simulink model "a1e2"  (R2020a)
settings: Solver=VariableStepAuto  StartTime=0.0  StopTime=50  RelTol=1e-3
settings Model: Creator=vivek vivian  LastModifiedBy=vivek vivian

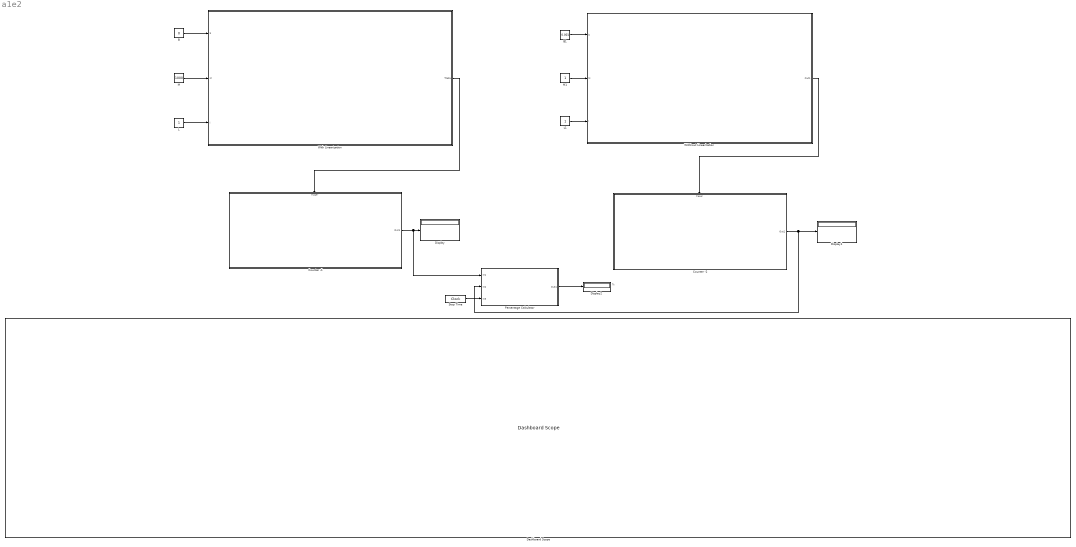
== system a1e2 ==
  note: %
  B : Constant  Value=0
  B1 : Constant  Value=0.001
  Counter -1 : Subsystem
  Counter -2 : Subsystem
  Dashboard Scope : DashboardScope
  Display : Display
  Display1 : Display
  Display2 : Display
  L : Constant
  L1 : Constant
  M : Constant  Value=1000
  M1 : Constant
  Percentage Calculator : Subsystem
  Stop Time : DigitalClock
  With Linearization : Subsystem
  Withhout Linearization : Subsystem
  wires:
  Counter -1/1(Out1) -> Percentage Calculator/1(In1), Display/1
  With Linearization/1(Theta) -> Counter -1/Trigger
  Counter -2/1(Out1) -> Percentage Calculator/2(In2), Display1/1
  Withhout Linearization/1(Out1) -> Counter -2/Trigger
  Percentage Calculator/1(Out1) -> Display2/1
  B/1 -> With Linearization/1(b)
  M/1 -> With Linearization/2(M)
  L/1 -> With Linearization/3(l)
  L1/1 -> Withhout Linearization/3(l)
  M1/1 -> Withhout Linearization/2(M)
  B1/1 -> Withhout Linearization/1(b)
  Stop Time/1 -> Percentage Calculator/3(In3)

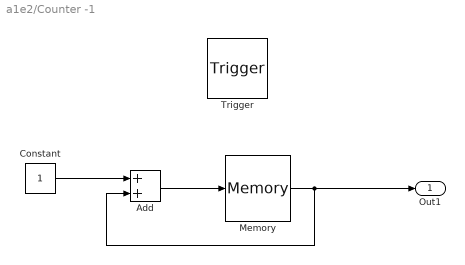
== system a1e2/Counter -1 ==
  Trigger : TriggerPort  VariantControl=Variant  PortDimensions=1
  Add : Sum
  Constant : Constant
  Memory : Memory  InheritSampleTime=on
  Out1 : Outport
  wires:
  Constant/1 -> Add/1
  Add/1 -> Memory/1
  Memory/1 -> Add/2, Out1/1

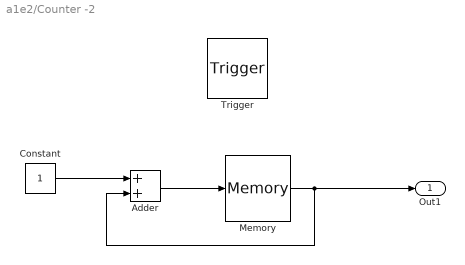
== system a1e2/Counter -2 ==
  Trigger : TriggerPort  VariantControl=Variant  PortDimensions=1
  Adder : Sum
  Constant : Constant
  Memory : Memory  InheritSampleTime=on
  Out1 : Outport
  wires:
  Constant/1 -> Adder/1
  Adder/1 -> Memory/1
  Memory/1 -> Adder/2, Out1/1

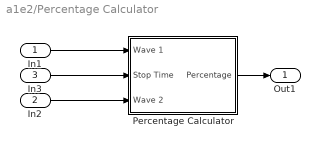
== system a1e2/Percentage Calculator ==
  In1 : Inport
  In2 : Inport  Port=2
  In3 : Inport  Port=3
  Percentage Calculator : Subsystem
  Out1 : Outport
  wires:
  In1/1 -> Percentage Calculator/1(Wave 1)
  In3/1 -> Percentage Calculator/2(Stop Time)
  In2/1 -> Percentage Calculator/3(Wave 2)
  Percentage Calculator/1(Percentage) -> Out1/1

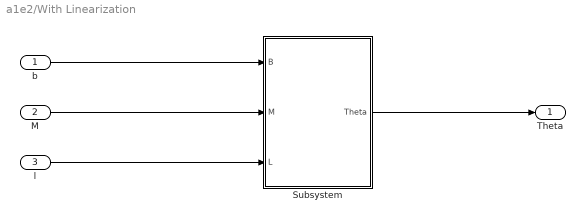
== system a1e2/With Linearization ==
  b : Inport
  M : Inport  Port=2
  l : Inport  Port=3
  Subsystem : Subsystem
  Theta : Outport
  wires:
  b/1 -> Subsystem/1(B)
  M/1 -> Subsystem/2(M)
  l/1 -> Subsystem/3(L)
  Subsystem/1(Theta) -> Theta/1

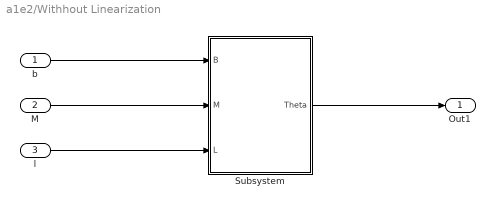
== system a1e2/Withhout Linearization ==
  b : Inport
  M : Inport  Port=2
  l : Inport  Port=3
  Subsystem : Subsystem
  Out1 : Outport
  wires:
  b/1 -> Subsystem/1(B)
  M/1 -> Subsystem/2(M)
  l/1 -> Subsystem/3(L)
  Subsystem/1(Theta) -> Out1/1

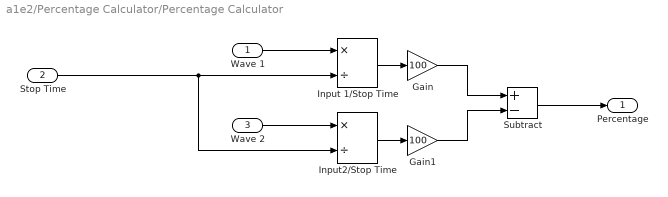
== system a1e2/Percentage Calculator/Percentage Calculator ==
  Wave 1 : Inport
  Stop Time : Inport  Port=2
  Wave 2 : Inport  Port=3
  Gain : Gain  Gain=100
  Gain1 : Gain  Gain=100
  Input 1/Stop Time : Product  Inputs=*/
  Input2/Stop Time : Product  Inputs=*/
  Subtract : Sum  Inputs=+-
  Percentage : Outport
  wires:
  Input 1/Stop Time/1 -> Gain/1
  Input2/Stop Time/1 -> Gain1/1
  Stop Time/1 -> Input2/Stop Time/2, Input 1/Stop Time/2
  Subtract/1 -> Percentage/1
  Gain1/1 -> Subtract/2
  Wave 2/1 -> Input2/Stop Time/1
  Wave 1/1 -> Input 1/Stop Time/1
  Gain/1 -> Subtract/1

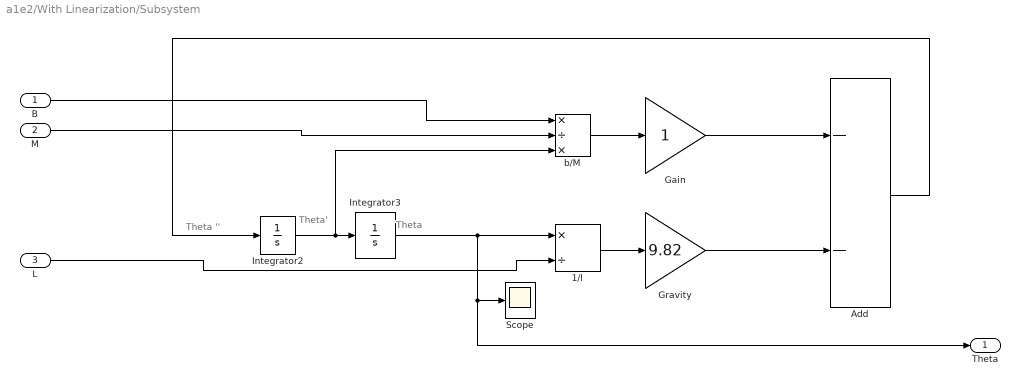
== system a1e2/With Linearization/Subsystem ==
  note: Theta
  note: Theta'
  note: Theta ''
  B : Inport
  M : Inport  Port=2
  L : Inport  Port=3
  1/l : Product  Inputs=*/
  Add : Sum  Inputs=--
  Gain : Gain
  Gravity : Gain  Gain=9.82
  Integrator2 : Integrator
  Integrator3 : Integrator  InitialCondition=pi/4
  Scope : Scope
  b/M : Product  Inputs=*/*
  Theta : Outport
  wires:
  Gravity/1 -> Add/2
  Integrator3/1 -> Theta/1, Scope/1, 1/l/1
  Add/1 -> Integrator2/1
  b/M/1 -> Gain/1
  Gain/1 -> Add/1
  1/l/1 -> Gravity/1
  B/1 -> b/M/1
  M/1 -> b/M/2
  Integrator2/1 -> b/M/3, Integrator3/1
  L/1 -> 1/l/2

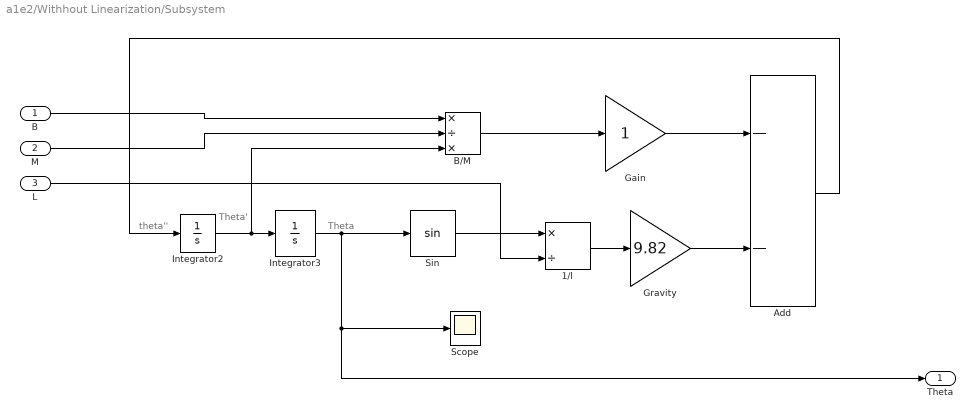
== system a1e2/Withhout Linearization/Subsystem ==
  note: Theta'
  note: theta''
  note: Theta
  B : Inport
  M : Inport  Port=2
  L : Inport  Port=3
  1/l : Product  Inputs=*/
  Add : Sum  Inputs=--
  B/M : Product  Inputs=*/*
  Gain : Gain
  Gravity : Gain  Gain=9.82
  Integrator2 : Integrator
  Integrator3 : Integrator  InitialCondition=pi/4
  Scope : Scope
  Sin : Trigonometry
  Theta : Outport
  wires:
  Integrator2/1 -> B/M/3, Integrator3/1
  Gain/1 -> Add/1
  Integrator3/1 -> Sin/1, Theta/1, Scope/1
  Sin/1 -> 1/l/1
  B/M/1 -> Gain/1
  Add/1 -> Integrator2/1
  L/1 -> 1/l/2
  Gravity/1 -> Add/2
  1/l/1 -> Gravity/1
  M/1 -> B/M/2
  B/1 -> B/M/1
